simulink model "ex2sim"  (R2025b)
settings: Solver=VariableStepAuto  StartTime=0.0  StopTime=10.0  RelTol=1e-3

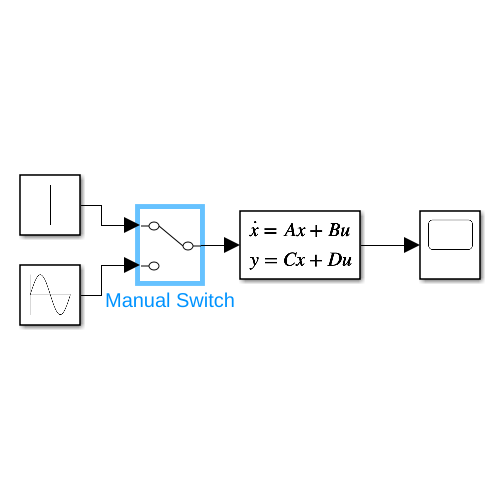
[thumbnail: Simulink's stored preview of the top-level diagram]
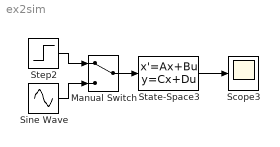
== system ex2sim ==
  Manual Switch : ManualSwitch
  Scope3 : Scope
      settings: ActiveDisplayYMinimum=-4.2235795853629385  ActiveDisplayYMaximum=6.3264990183680068  DataLoggingVariableName=ScopeData3
  Sine Wave : Sin  Frequency=2*3.14  SampleTime=0
  State-Space3 : StateSpace  A=[0, 1, 0; 0, 0, 1; -6, -11, -6]  B=[1; 1; 1]  C=[1, 1, 0]  InitialCondition=[1; 0.5; -0.5]
  Step2 : Step  SampleTime=0
  wires:
  State-Space3/1 -> Scope3/1
  Manual Switch/1 -> State-Space3/1
  Sine Wave/1 -> Manual Switch/2
  Step2/1 -> Manual Switch/1
